simulink model "rowFaz_schemat"  (R2024b)
settings: Solver=VariableStepAuto  StartTime=0.0  StopTime=10.0  RelTol=1e-3
values from neighbouring files (symbols this model uses):
  czas_skok = 1    [ksi0.m]    (also in ksi02.m; ksi2.m; ksiMinus02.m; ksiMinus2.m)
  dU = 0    [ksi0.m]    (also in ksi02.m; ksi2.m; ksiMinus02.m; ksiMinus2.m)
  ksi = 0    [ksi0.m]    (also in ksi02.m = 0.2; ksi2.m = 2; ksiMinus02.m = -0.2; ksiMinus2.m = -2)
  U0 = 0    [ksi0.m]    (also in ksi02.m; ksi2.m; ksiMinus02.m; ksiMinus2.m)
  wn = 5    [ksi0.m]    (also in ksi02.m; ksi2.m; ksiMinus02.m; ksiMinus2.m)
  X0 = [1, -3, -2]    [ksi0.m]    (also in ksi02.m; ksi2.m = [1, -3, -5, 5, 2, -2]; ksiMinus02.m; ksiMinus2.m = [1, -3])
  Xp0 = [5, 6, -5]    [ksi0.m]    (also in ksi02.m; ksi2.m = [5, 6, 4, -5, -7, -6]; ksiMinus02.m; ksiMinus2.m = [5, -6])
settings Model: Creator=Michal  LastModifiedBy=Michal
settings DataIOCC: ReturnWorkspaceOutputs=off

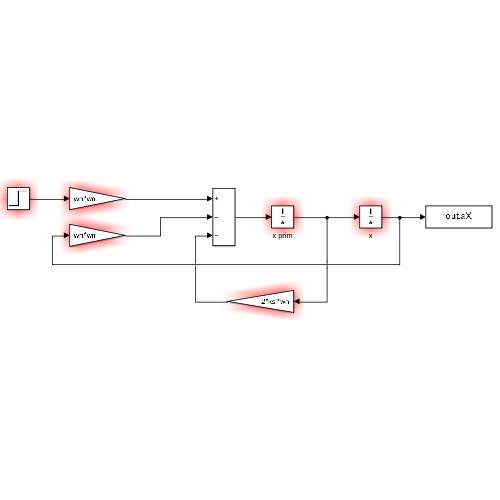
[thumbnail: Simulink's stored preview of the top-level diagram]
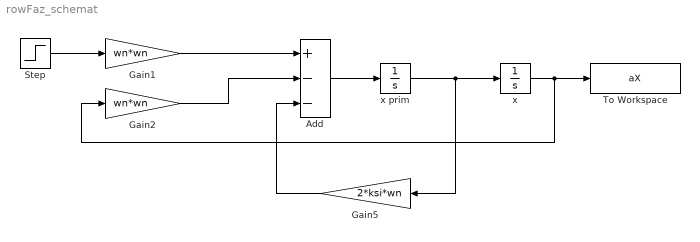
== system rowFaz_schemat ==
  Add : Sum  Inputs=+--
  Gain1 : Gain  Gain=wn*wn
  Gain2 : Gain  Gain=wn*wn
  Gain5 : Gain  Gain=2*ksi*wn
  Step : Step  Time=czas_skok  Before=U0  After=U0+dU  SampleTime=0
  To Workspace : ToWorkspace  VariableName=aX  SampleTime=-1
  x : Integrator  InitialCondition=X0
  x prim : Integrator  InitialCondition=Xp0
  wires:
  x prim/1 -> Gain5/1, x/1
  Step/1 -> Gain1/1
  Add/1 -> x prim/1
  x/1 -> Gain2/1, To Workspace/1
  Gain5/1 -> Add/3
  Gain2/1 -> Add/2
  Gain1/1 -> Add/1
